simulink model "cube_controller"  (R2023b)
settings: Solver=VariableStepAuto  StartTime=0.0  StopTime=10.0  RelTol=1e-3
settings Model: Creator=charl  LastModifiedBy=charl

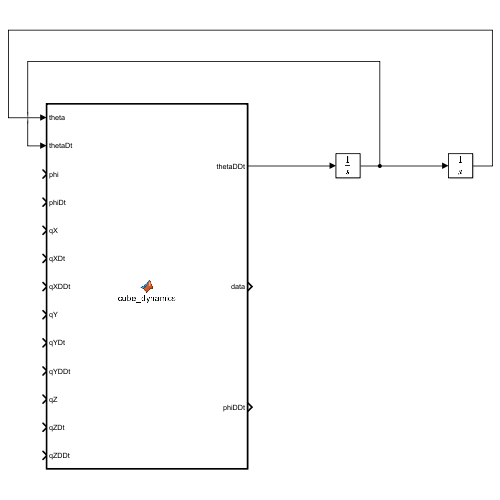
[thumbnail: Simulink's stored preview of the top-level diagram]
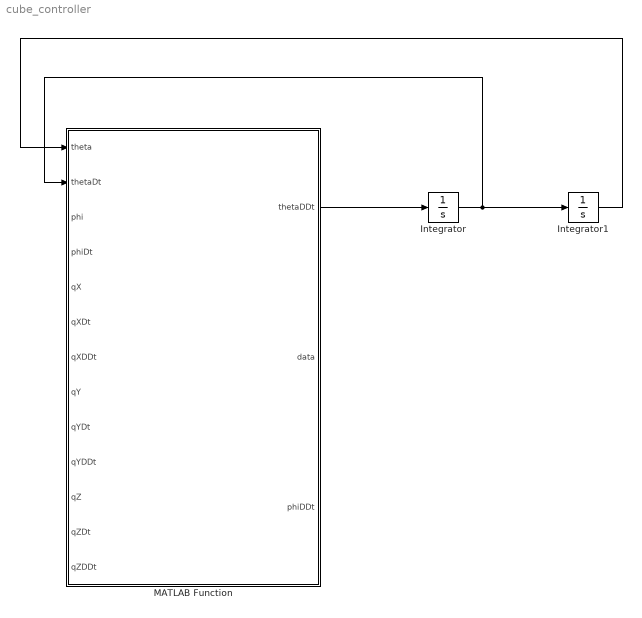
== system cube_controller ==
  Integrator : Integrator
  Integrator1 : Integrator
  MATLAB Function : MATLAB Function  TreatAsAtomicUnit=on
  wires:
  MATLAB Function/1(thetaDDt) -> Integrator/1
  Integrator/1 -> Integrator1/1, MATLAB Function/2(thetaDt)
  Integrator1/1 -> MATLAB Function/1(theta)

== matlab function cube_controller/MATLAB Function ==
  data: theta input; thetaDt input; thetaDDt output; data output; phi input; phiDt input; qX input; qXDt input; qXDDt input; qY input; qYDt input; qYDDt input; qZ input; qZDt input; qZDDt input; phiDDt output
function [thetaDDt, data, phiDDt]= cube_dynamics(theta, thetaDt, phi, phiDt, qX, qXDt, qXDDt, qY, qYDt, qYDDt, qZ, qZDt, qZDDt)


thetaDDt = -((RXIXY*sin(theta)*cos(phi+qX)+(RZIXY*cos(qZ)-RZIYY*sin(qZ))*(sin(qZ)*cos(theta)+sin(theta)*cos(phi)*cos(qZ))-RXIXZ*sin(  ...
theta)*sin(phi+qX)-(CIXX+RXIXX+mR*RCMZ^2+2*mR*(RCMY^2+1.5*RCMX^2))*cos(theta)-(RYIXZ*cos(qY)+RYIZZ*sin(qY))*(sin(qY)*cos(theta)+sin(  ...
phi)*sin(theta)*cos(qY))-(RYIXX*cos(qY)+RYIXZ*sin(qY))*(cos(qY)*cos(theta)-sin(phi)*sin(qY)*sin(theta))-(RZIXX*cos(qZ)-RZIXY*sin(  ...
qZ))*(cos(qZ)*cos(theta)-sin(qZ)*sin(theta)*cos(phi))-sin(phi)*sin(theta)*(CIXZ+mR*RCMX*RCMY+mR*RCMX^2+mR*RCMY*RCMZ+RZIXZ*cos(qZ)-  ...
RZIYZ*sin(qZ))-sin(theta)*cos(phi)*(mR*RCMX*RCMY+mR*RCMX*RCMZ+mR*RCMY*RCMZ-CIXY-RYIXY*cos(qY)-RYIYZ*sin(qY)))*(g*((mC*CCMZ+mR*RCMX+  ...
mR*RCMY+mR*RCMZ)*cos(theta)-(mC*CCMY+mR*RCMY+2*mR*RCMX)*sin(phi)*sin(theta)-(mC*CCMX+mR*RCMX+mR*RCMY+mR*RCMZ)*sin(theta)*cos(phi))+  ...
cos(phi+qX)*(2*RXIYZ*cos(phi+qX)*thetaDt*(phiDt+qXDt)+(phiDt+qXDt)*(RXIXY*(phiDt+qXDt)+2*RXIYY*sin(phi+qX)*thetaDt)+RXIXZ*qXDDt)+  ...
sin(qY)*cos(phi)*(RYIXX*sin(qY)*phiDt*qYDt+2*RYIXX*cos(phi)*cos(qY)*qYDt*thetaDt+2*RYIXZ*sin(qY)*cos(phi)*qYDt*thetaDt+4*RYIXZ*sin(  ...
phi)*cos(qY)*phiDt*thetaDt-4*RYIXZ*cos(qY)*phiDt*qYDt-2*RYIXY*cos(phi)*phiDt*thetaDt-2*RYIXX*sin(phi)*sin(qY)*phiDt*thetaDt-qYDt*(  ...
RYIYZ*qYDt+RYIZZ*sin(qY)*phiDt+2*RYIYZ*sin(phi)*thetaDt+2*RYIZZ*cos(phi)*cos(qY)*thetaDt)-RYIXY*qYDDt)-sin(phi+qX)*(2*RXIYZ*sin(phi+  ...
qX)*thetaDt*(phiDt+qXDt)+(phiDt+qXDt)*(RXIXZ*(phiDt+qXDt)+2*RXIZZ*cos(phi+qX)*thetaDt)-RXIXY*qXDDt)-cos(phi)*cos(qY)*(qYDt*(  ...
RYIXY*qYDt+RYIXX*cos(qY)*phiDt)+2*RYIXZ*cos(phi)*cos(qY)*qYDt*thetaDt-RYIZZ*cos(qY)*phiDt*qYDt-RYIYZ*qYDDt)-sin(phi)*cos(qZ)*(  ...
RZIYY*cos(qZ)*phiDt*qZDt+2*RZIXY*sin(qZ)*phiDt*qZDt+RZIYY*sin(phi)*sin(qZ)*qZDt*thetaDt-RZIXY*sin(phi)*cos(qZ)*qZDt*thetaDt-  ...
RZIYY*cos(phi)*cos(qZ)*phiDt*thetaDt-(qZDt+cos(phi)*thetaDt)*(RZIXZ*qZDt+RZIXX*cos(qZ)*phiDt+RZIXZ*cos(phi)*thetaDt+RZIXX*sin(phi)*  ...
sin(qZ)*thetaDt+RZIXY*sin(phi)*cos(qZ)*thetaDt)-RZIYZ*qZDDt)-sin(phi)*sin(qZ)*(RZIXX*sin(qZ)*phiDt*qZDt+RZIXY*sin(phi)*sin(qZ)*qZDt*  ...
thetaDt-2*RZIXY*cos(phi)*cos(qZ)*phiDt*thetaDt-RZIXX*sin(phi)*cos(qZ)*qZDt*thetaDt-RZIXX*sin(qZ)*cos(phi)*phiDt*thetaDt-(qZDt+cos(  ...
phi)*thetaDt)*(RZIYY*sin(qZ)*phiDt-RZIYZ*qZDt-2*RZIXY*cos(qZ)*phiDt-RZIYZ*cos(phi)*thetaDt-RZIXY*sin(phi)*sin(qZ)*thetaDt-RZIYY*sin(  ...
phi)*cos(qZ)*thetaDt)-RZIXZ*qZDDt)-sin(phi)*(2*RYIXY*cos(phi)*cos(qY)*qYDt*thetaDt+cos(qY)*phiDt*(RYIXZ*cos(qY)*phiDt+RYIZZ*sin(qY)*  ...
phiDt+2*RYIYZ*sin(phi)*thetaDt+2*RYIZZ*cos(phi)*cos(qY)*thetaDt)-2*CIYY*cos(phi)*phiDt*thetaDt-2*RYIYY*cos(phi)*phiDt*thetaDt-2*  ...
RYIXY*sin(phi)*sin(qY)*phiDt*thetaDt-sin(qY)*(RYIXX*cos(qY)+RYIXZ*sin(qY))*phiDt^2-phiDt*(RZIYZ*sin(qZ)*phiDt-CIXZ*phiDt-RZIZZ*qZDt-  ...
2*CIYZ*sin(phi)*thetaDt-2*CIZZ*cos(phi)*thetaDt-2*RZIZZ*cos(phi)*thetaDt-RZIXZ*cos(qZ)*phiDt-2*RZIXZ*sin(phi)*sin(qZ)*thetaDt-2*  ...
RZIYZ*sin(phi)*cos(qZ)*thetaDt-mR*RCMX*(RCMX*phiDt+4*RCMY*sin(phi)*thetaDt)-mR*(RCMY*RCMZ*phiDt-2*RCMX^2*cos(phi)*thetaDt)-mR*(RCMX*  ...
RCMY*phiDt+2*RCMZ*(RCMX*sin(phi)+RCMZ*cos(phi))*thetaDt))-RYIYY*qYDDt)-cos(phi)*(RZIXZ*sin(qZ)*phiDt*qZDt+RZIYZ*cos(qZ)*phiDt*qZDt+  ...
RZIYZ*sin(phi)*sin(qZ)*qZDt*thetaDt+(cos(qZ)*phiDt+sin(phi)*sin(qZ)*thetaDt)*(RZIYY*sin(qZ)*phiDt-RZIYZ*qZDt-RZIXY*cos(qZ)*phiDt-  ...
RZIYZ*cos(phi)*thetaDt-RZIXY*sin(phi)*sin(qZ)*thetaDt-RZIYY*sin(phi)*cos(qZ)*thetaDt)+(sin(qZ)*phiDt-sin(phi)*cos(qZ)*thetaDt)*(  ...
RZIXY*sin(qZ)*phiDt-RZIXZ*qZDt-RZIXX*cos(qZ)*phiDt-RZIXZ*cos(phi)*thetaDt-RZIXX*sin(phi)*sin(qZ)*thetaDt-RZIXY*sin(phi)*cos(qZ)*  ...
thetaDt)-2*CIYZ*cos(phi)*phiDt*thetaDt-RZIXZ*sin(phi)*cos(qZ)*qZDt*thetaDt-RZIXZ*sin(qZ)*cos(phi)*phiDt*thetaDt-RZIYZ*cos(phi)*cos(  ...
qZ)*phiDt*thetaDt-phiDt*(CIXY*phiDt+RYIYY*qYDt+RYIXY*cos(qY)*phiDt+RYIYZ*sin(qY)*phiDt+2*RYIYZ*cos(phi)*cos(qY)*thetaDt-mR*RCMX*RCMY*  ...
phiDt-mR*RCMX*(RCMZ*phiDt-4*RCMY*cos(phi)*thetaDt)-mR*RCMZ*(RCMY*phiDt-2*RCMX*cos(phi)*thetaDt))-RZIZZ*qZDDt))+(RXIXY*sin(phi+qX)+  ...
RXIXZ*cos(phi+qX)+cos(phi)*cos(qY)*(RYIXZ*cos(qY)+RYIZZ*sin(qY))+sin(phi)*sin(qZ)*(RZIXX*cos(qZ)-RZIXY*sin(qZ))+sin(phi)*cos(qZ)*(  ...
RZIXY*cos(qZ)-RZIYY*sin(qZ))+cos(phi)*(CIXZ+mR*RCMX*RCMY+mR*RCMX^2+mR*RCMY*RCMZ+RZIXZ*cos(qZ)-RZIYZ*sin(qZ))-sin(qY)*cos(phi)*(  ...
RYIXX*cos(qY)+RYIXZ*sin(qY))-sin(phi)*(mR*RCMX*RCMY+mR*RCMX*RCMZ+mR*RCMY*RCMZ-CIXY-RYIXY*cos(qY)-RYIYZ*sin(qY)))*(g*((mC*CCMY+mR*  ...
RCMY+2*mR*RCMX)*cos(phi)-(mC*CCMX+mR*RCMX+mR*RCMY+mR*RCMZ)*sin(phi))+sin(theta)*thetaDt*(mR*RCMZ*(RCMX*sin(phi)-RCMY*cos(phi))*  ...
thetaDt-CIXX*phiDt-RXIXX*(phiDt+qXDt)-CIXY*sin(phi)*thetaDt-CIXZ*cos(phi)*thetaDt-RXIXY*sin(phi+qX)*thetaDt-RXIXZ*cos(phi+qX)*  ...
thetaDt-2*mR*(RCMY^2+1.5*RCMX^2)*phiDt-mR*RCMX*(RCMX*cos(phi)-RCMY*sin(phi))*thetaDt-mR*(RCMZ^2*phiDt+RCMY*(RCMX*cos(phi)-RCMZ*sin(  ...
phi))*thetaDt))+sin(theta)*cos(phi+qX)*(4*RXIYZ*sin(phi+qX)*thetaDt*(phiDt+qXDt)+(phiDt+qXDt)*(RXIXZ*(phiDt+qXDt)+RXIZZ*cos(phi+qX)*  ...
thetaDt)-RXIYY*cos(phi+qX)*thetaDt*(phiDt+qXDt)-RXIXY*qXDDt)+(sin(qZ)*cos(theta)+sin(theta)*cos(phi)*cos(qZ))*(RZIXY*sin(qZ)*  ...
phiDt*qZDt+RZIYY*cos(qZ)*phiDt*qZDt+RZIYZ*sin(phi)*phiDt*thetaDt+RZIYY*sin(phi)*sin(qZ)*qZDt*thetaDt+(qZDt+cos(phi)*thetaDt)*(  ...
RZIXY*sin(qZ)*phiDt-RZIXZ*qZDt-RZIXX*cos(qZ)*phiDt-RZIXZ*cos(phi)*thetaDt-RZIXX*sin(phi)*sin(qZ)*thetaDt-RZIXY*sin(phi)*cos(qZ)*  ...
thetaDt)-RZIXY*sin(phi)*cos(qZ)*qZDt*thetaDt-RZIXY*sin(qZ)*cos(phi)*phiDt*thetaDt-RZIYY*cos(phi)*cos(qZ)*phiDt*thetaDt-RZIYZ*  ...
qZDDt)+sin(theta)*cos(phi)*(RYIXY*sin(qY)*phiDt*qYDt+RYIXY*cos(phi)*cos(qY)*qYDt*thetaDt+RYIYZ*sin(qY)*cos(phi)*qYDt*thetaDt+(sin(  ...
qY)*phiDt+cos(phi)*cos(qY)*thetaDt)*(RYIXX*sin(qY)*cos(phi)*thetaDt-RYIXY*qYDt-RYIXX*cos(qY)*phiDt-RYIXY*sin(phi)*thetaDt-RYIXZ*sin(  ...
qY)*phiDt-RYIXZ*cos(phi)*cos(qY)*thetaDt)-CIYY*cos(phi)*phiDt*thetaDt-RYIYY*cos(phi)*phiDt*thetaDt-RYIYZ*cos(qY)*phiDt*qYDt-(cos(  ...
qY)*phiDt-sin(qY)*cos(phi)*thetaDt)*(RYIXZ*sin(qY)*cos(phi)*thetaDt-RYIYZ*qYDt-RYIXZ*cos(qY)*phiDt-RYIYZ*sin(phi)*thetaDt-RYIZZ*sin(  ...
qY)*phiDt-RYIZZ*cos(phi)*cos(qY)*thetaDt)-phiDt*(RZIYZ*sin(qZ)*phiDt-CIXZ*phiDt-RZIZZ*qZDt-mR*RCMX^2*phiDt-CIZZ*cos(phi)*thetaDt-  ...
RZIXZ*cos(qZ)*phiDt-RZIZZ*cos(phi)*thetaDt-mR*(RCMX*RCMY*phiDt+RCMZ^2*cos(phi)*thetaDt)-mR*(RCMY*RCMZ*phiDt-RCMX^2*cos(phi)*  ...
thetaDt))-RYIYY*qYDDt)-sin(theta)*sin(phi+qX)*(RXIZZ*sin(phi+qX)*thetaDt*(phiDt+qXDt)-(phiDt+qXDt)*(RXIXY*(phiDt+qXDt)+RXIYY*sin(  ...
phi+qX)*thetaDt)-RXIXZ*qXDDt)-(sin(qY)*cos(theta)+sin(phi)*sin(theta)*cos(qY))*(RYIXZ*sin(qY)*phiDt*qYDt+RYIXZ*cos(phi)*cos(qY)*qYDt*  ...
thetaDt+RYIZZ*sin(phi)*cos(qY)*phiDt*thetaDt+RYIZZ*sin(qY)*cos(phi)*qYDt*thetaDt-RYIYZ*cos(phi)*phiDt*thetaDt-RYIZZ*cos(qY)*  ...
phiDt*qYDt-RYIXZ*sin(phi)*sin(qY)*phiDt*thetaDt-(qYDt+sin(phi)*thetaDt)*(RYIXX*sin(qY)*cos(phi)*thetaDt-RYIXY*qYDt-RYIXX*cos(qY)*  ...
phiDt-RYIXY*sin(phi)*thetaDt-RYIXZ*sin(qY)*phiDt-RYIXZ*cos(phi)*cos(qY)*thetaDt)-RYIYZ*qYDDt)-(cos(qY)*cos(theta)-sin(phi)*sin(qY)*  ...
sin(theta))*(RYIXX*sin(qY)*phiDt*qYDt+RYIXX*cos(phi)*cos(qY)*qYDt*thetaDt+RYIXZ*sin(phi)*cos(qY)*phiDt*thetaDt+RYIXZ*sin(qY)*cos(  ...
phi)*qYDt*thetaDt+(qYDt+sin(phi)*thetaDt)*(RYIXZ*sin(qY)*cos(phi)*thetaDt-RYIYZ*qYDt-RYIXZ*cos(qY)*phiDt-RYIYZ*sin(phi)*thetaDt-  ...
RYIZZ*sin(qY)*phiDt-RYIZZ*cos(phi)*cos(qY)*thetaDt)-RYIXY*cos(phi)*phiDt*thetaDt-RYIXZ*cos(qY)*phiDt*qYDt-RYIXX*sin(phi)*sin(qY)*  ...
phiDt*thetaDt-RYIXY*qYDDt)-(cos(qZ)*cos(theta)-sin(qZ)*sin(theta)*cos(phi))*(RZIXX*sin(qZ)*phiDt*qZDt+RZIXY*cos(qZ)*phiDt*qZDt+  ...
RZIXZ*sin(phi)*phiDt*thetaDt+RZIXY*sin(phi)*sin(qZ)*qZDt*thetaDt-RZIXX*sin(phi)*cos(qZ)*qZDt*thetaDt-RZIXX*sin(qZ)*cos(phi)*  ...
phiDt*thetaDt-RZIXY*cos(phi)*cos(qZ)*phiDt*thetaDt-(qZDt+cos(phi)*thetaDt)*(RZIYY*sin(qZ)*phiDt-RZIYZ*qZDt-RZIXY*cos(qZ)*phiDt-  ...
RZIYZ*cos(phi)*thetaDt-RZIXY*sin(phi)*sin(qZ)*thetaDt-RZIYY*sin(phi)*cos(qZ)*thetaDt)-RZIXZ*qZDDt)-cos(theta)*(sin(phi)*thetaDt*(  ...
RZIYZ*sin(qZ)*phiDt-RZIZZ*qZDt-CIYZ*sin(phi)*thetaDt-CIZZ*cos(phi)*thetaDt-RZIXZ*cos(qZ)*phiDt-RZIZZ*cos(phi)*thetaDt-2*mR*RCMX*RCMY*  ...
sin(phi)*thetaDt-RZIXZ*sin(phi)*sin(qZ)*thetaDt-RZIYZ*sin(phi)*cos(qZ)*thetaDt-mR*RCMZ*(RCMX*sin(phi)+RCMZ*cos(phi))*thetaDt)-(sin(  ...
phi+qX)*(RXIYZ*sin(phi+qX)+RXIZZ*cos(phi+qX))-cos(phi+qX)*(RXIYY*sin(phi+qX)+RXIYZ*cos(phi+qX)))*thetaDt^2-cos(phi)*thetaDt*(  ...
RYIXY*sin(qY)*cos(phi)*thetaDt-RYIYY*qYDt-CIYY*sin(phi)*thetaDt-CIYZ*cos(phi)*thetaDt-RYIXY*cos(qY)*phiDt-RYIYY*sin(phi)*thetaDt-  ...
RYIYZ*sin(qY)*phiDt-2*mR*RCMX*RCMY*cos(phi)*thetaDt-mR*RCMX*RCMZ*cos(phi)*thetaDt-mR*RCMX^2*sin(phi)*thetaDt-RYIYZ*cos(phi)*cos(qY)*  ...
thetaDt)-RXIXX*qXDDt)-sin(phi)*sin(theta)*(CIZZ*sin(phi)*phiDt*thetaDt+RZIXZ*sin(qZ)*phiDt*qZDt+RZIYZ*cos(qZ)*phiDt*qZDt+RZIZZ*sin(  ...
phi)*phiDt*thetaDt+mR*RCMZ^2*sin(phi)*phiDt*thetaDt+RZIYZ*sin(phi)*sin(qZ)*qZDt*thetaDt+(cos(qZ)*phiDt+sin(phi)*sin(qZ)*thetaDt)*(  ...
RZIYY*sin(qZ)*phiDt-RZIYZ*qZDt-RZIXY*cos(qZ)*phiDt-RZIYZ*cos(phi)*thetaDt-RZIXY*sin(phi)*sin(qZ)*thetaDt-RZIYY*sin(phi)*cos(qZ)*  ...
thetaDt)+(sin(qZ)*phiDt-sin(phi)*cos(qZ)*thetaDt)*(RZIXY*sin(qZ)*phiDt-RZIXZ*qZDt-RZIXX*cos(qZ)*phiDt-RZIXZ*cos(phi)*thetaDt-  ...
RZIXX*sin(phi)*sin(qZ)*thetaDt-RZIXY*sin(phi)*cos(qZ)*thetaDt)-4*CIYZ*cos(phi)*phiDt*thetaDt-2*RZIXZ*sin(qZ)*cos(phi)*phiDt*  ...
thetaDt-2*RZIYZ*cos(phi)*cos(qZ)*phiDt*thetaDt-RZIXZ*sin(phi)*cos(qZ)*qZDt*thetaDt-phiDt*(CIXY*phiDt+RYIYY*qYDt+CIYY*sin(phi)*  ...
thetaDt+RYIXY*cos(qY)*phiDt+RYIYY*sin(phi)*thetaDt+RYIYZ*sin(qY)*phiDt+2*RYIYZ*cos(phi)*cos(qY)*thetaDt-2*RYIXY*sin(qY)*cos(phi)*  ...
thetaDt-mR*RCMX*(RCMY*phiDt-RCMX*sin(phi)*thetaDt)-mR*RCMX*(RCMZ*phiDt-8*RCMY*cos(phi)*thetaDt)-mR*RCMZ*(RCMY*phiDt-4*RCMX*cos(phi)*  ...
thetaDt))-RZIZZ*qZDDt)))/((2*mR*RCMY^2+mR*(RCMX^2+RCMZ^2)+RXIYY*sin(phi+qX)^2+RYIZZ*cos(phi)^2*cos(qY)^2+RZIXX*sin(phi)^2*sin(qZ)^2+  ...
cos(phi+qX)*(RXIZZ*cos(phi+qX)+2*RXIYZ*sin(phi+qX))+cos(qZ)*sin(phi)^2*(RZIYY*cos(qZ)+2*RZIXY*sin(qZ))+sin(qY)*cos(phi)*(RYIXX*sin(  ...
qY)*cos(phi)-2*RYIXY*sin(phi)-2*RYIXZ*cos(phi)*cos(qY))+cos(phi)*(CIZZ*cos(phi)+RZIZZ*cos(phi)+mR*RCMX^2*cos(phi)+mR*RCMZ^2*cos(phi)+  ...
2*RZIXZ*sin(phi)*sin(qZ)+2*RZIYZ*sin(phi)*cos(qZ))+sin(phi)*(CIYY*sin(phi)+RYIYY*sin(phi)+2*CIYZ*cos(phi)+2*mR*RCMX*RCMZ*cos(phi)+  ...
2*mR*RCMX^2*sin(phi)+4*mR*RCMX*RCMY*cos(phi)+2*RYIYZ*cos(phi)*cos(qY)))*(RXIXY*sin(theta)*cos(phi+qX)+(RZIXY*cos(qZ)-RZIYY*sin(qZ))*(  ...
sin(qZ)*cos(theta)+sin(theta)*cos(phi)*cos(qZ))-RXIXZ*sin(theta)*sin(phi+qX)-(CIXX+RXIXX+mR*RCMZ^2+2*mR*(RCMY^2+1.5*RCMX^2))*cos(  ...
theta)-(RYIXZ*cos(qY)+RYIZZ*sin(qY))*(sin(qY)*cos(theta)+sin(phi)*sin(theta)*cos(qY))-(RYIXX*cos(qY)+RYIXZ*sin(qY))*(cos(qY)*cos(  ...
theta)-sin(phi)*sin(qY)*sin(theta))-(RZIXX*cos(qZ)-RZIXY*sin(qZ))*(cos(qZ)*cos(theta)-sin(qZ)*sin(theta)*cos(phi))-sin(phi)*sin(  ...
theta)*(CIXZ+mR*RCMX*RCMY+mR*RCMX^2+mR*RCMY*RCMZ+RZIXZ*cos(qZ)-RZIYZ*sin(qZ))-sin(theta)*cos(phi)*(mR*RCMX*RCMY+mR*RCMX*RCMZ+mR*RCMY*  ...
RCMZ-CIXY-RYIXY*cos(qY)-RYIYZ*sin(qY)))+(RXIXY*sin(phi+qX)+RXIXZ*cos(phi+qX)+cos(phi)*cos(qY)*(RYIXZ*cos(qY)+RYIZZ*sin(qY))+sin(phi)*  ...
sin(qZ)*(RZIXX*cos(qZ)-RZIXY*sin(qZ))+sin(phi)*cos(qZ)*(RZIXY*cos(qZ)-RZIYY*sin(qZ))+cos(phi)*(CIXZ+mR*RCMX*RCMY+mR*RCMX^2+mR*RCMY*  ...
RCMZ+RZIXZ*cos(qZ)-RZIYZ*sin(qZ))-sin(qY)*cos(phi)*(RYIXX*cos(qY)+RYIXZ*sin(qY))-sin(phi)*(mR*RCMX*RCMY+mR*RCMX*RCMZ+mR*RCMY*RCMZ-  ...
CIXY-RYIXY*cos(qY)-RYIYZ*sin(qY)))*(sin(theta)*sin(phi+qX)*(RXIYZ*sin(phi+qX)+RXIZZ*cos(phi+qX))+(cos(qZ)*cos(theta)-sin(qZ)*sin(  ...
theta)*cos(phi))*(RZIXZ*cos(phi)+RZIXX*sin(phi)*sin(qZ)+RZIXY*sin(phi)*cos(qZ))+sin(theta)*cos(phi)*(RYIXY*sin(qY)*cos(phi)-CIYY*  ...
sin(phi)-CIYZ*cos(phi)-RYIYY*sin(phi)-2*mR*RCMX*RCMY*cos(phi)-mR*RCMX*RCMZ*cos(phi)-RYIYZ*cos(phi)*cos(qY))+cos(theta)*(CIXY*sin(  ...
phi)+CIXZ*cos(phi)+RXIXY*sin(phi+qX)+RXIXZ*cos(phi+qX)+mR*RCMX*(RCMX*cos(phi)-RCMY*sin(phi))+mR*RCMY*(RCMX*cos(phi)-RCMZ*sin(phi))-  ...
mR*RCMZ*(RCMX*sin(phi)-RCMY*cos(phi)))-sin(theta)*cos(phi+qX)*(RXIYY*sin(phi+qX)+RXIYZ*cos(phi+qX))-(sin(qZ)*cos(theta)+sin(  ...
theta)*cos(phi)*cos(qZ))*(RZIYZ*cos(phi)+RZIXY*sin(phi)*sin(qZ)+RZIYY*sin(phi)*cos(qZ))-(sin(qY)*cos(theta)+sin(phi)*sin(theta)*cos(  ...
qY))*(RYIXZ*sin(qY)*cos(phi)-RYIYZ*sin(phi)-RYIZZ*cos(phi)*cos(qY))-(cos(qY)*cos(theta)-sin(phi)*sin(qY)*sin(theta))*(RYIXX*sin(qY)*  ...
cos(phi)-RYIXY*sin(phi)-RYIXZ*cos(phi)*cos(qY))-sin(phi)*sin(theta)*(mR*RCMX^2*cos(phi)-CIYZ*sin(phi)-CIZZ*cos(phi)-RZIZZ*cos(phi)-  ...
2*mR*RCMX*RCMY*sin(phi)-RZIXZ*sin(phi)*sin(qZ)-RZIYZ*sin(phi)*cos(qZ)-mR*RCMZ*(RCMX*sin(phi)+RCMZ*cos(phi)))));
phiDDt = -((sin(theta)*sin(phi+qX)*(RXIYZ*sin(phi+qX)+RXIZZ*cos(phi+qX))+(cos(qZ)*cos(theta)-sin(qZ)*sin(theta)*cos(phi))*(RZIXZ*  ...
cos(phi)+RZIXX*sin(phi)*sin(qZ)+RZIXY*sin(phi)*cos(qZ))+sin(theta)*cos(phi)*(RYIXY*sin(qY)*cos(phi)-CIYY*sin(phi)-CIYZ*cos(phi)-  ...
RYIYY*sin(phi)-2*mR*RCMX*RCMY*cos(phi)-mR*RCMX*RCMZ*cos(phi)-RYIYZ*cos(phi)*cos(qY))+cos(theta)*(CIXY*sin(phi)+CIXZ*cos(phi)+  ...
RXIXY*sin(phi+qX)+RXIXZ*cos(phi+qX)+mR*RCMX*(RCMX*cos(phi)-RCMY*sin(phi))+mR*RCMY*(RCMX*cos(phi)-RCMZ*sin(phi))-mR*RCMZ*(RCMX*sin(  ...
phi)-RCMY*cos(phi)))-sin(theta)*cos(phi+qX)*(RXIYY*sin(phi+qX)+RXIYZ*cos(phi+qX))-(sin(qZ)*cos(theta)+sin(theta)*cos(phi)*cos(qZ))*(  ...
RZIYZ*cos(phi)+RZIXY*sin(phi)*sin(qZ)+RZIYY*sin(phi)*cos(qZ))-(sin(qY)*cos(theta)+sin(phi)*sin(theta)*cos(qY))*(RYIXZ*sin(qY)*cos(  ...
phi)-RYIYZ*sin(phi)-RYIZZ*cos(phi)*cos(qY))-(cos(qY)*cos(theta)-sin(phi)*sin(qY)*sin(theta))*(RYIXX*sin(qY)*cos(phi)-RYIXY*sin(phi)-  ...
RYIXZ*cos(phi)*cos(qY))-sin(phi)*sin(theta)*(mR*RCMX^2*cos(phi)-CIYZ*sin(phi)-CIZZ*cos(phi)-RZIZZ*cos(phi)-2*mR*RCMX*RCMY*sin(phi)-  ...
RZIXZ*sin(phi)*sin(qZ)-RZIYZ*sin(phi)*cos(qZ)-mR*RCMZ*(RCMX*sin(phi)+RCMZ*cos(phi))))*(g*((mC*CCMZ+mR*RCMX+mR*RCMY+mR*RCMZ)*cos(  ...
theta)-(mC*CCMY+mR*RCMY+2*mR*RCMX)*sin(phi)*sin(theta)-(mC*CCMX+mR*RCMX+mR*RCMY+mR*RCMZ)*sin(theta)*cos(phi))+cos(phi+qX)*(2*  ...
RXIYZ*cos(phi+qX)*thetaDt*(phiDt+qXDt)+(phiDt+qXDt)*(RXIXY*(phiDt+qXDt)+2*RXIYY*sin(phi+qX)*thetaDt)+RXIXZ*qXDDt)+sin(qY)*cos(phi)*(  ...
RYIXX*sin(qY)*phiDt*qYDt+2*RYIXX*cos(phi)*cos(qY)*qYDt*thetaDt+2*RYIXZ*sin(qY)*cos(phi)*qYDt*thetaDt+4*RYIXZ*sin(phi)*cos(qY)*  ...
phiDt*thetaDt-4*RYIXZ*cos(qY)*phiDt*qYDt-2*RYIXY*cos(phi)*phiDt*thetaDt-2*RYIXX*sin(phi)*sin(qY)*phiDt*thetaDt-qYDt*(RYIYZ*qYDt+  ...
RYIZZ*sin(qY)*phiDt+2*RYIYZ*sin(phi)*thetaDt+2*RYIZZ*cos(phi)*cos(qY)*thetaDt)-RYIXY*qYDDt)-sin(phi+qX)*(2*RXIYZ*sin(phi+qX)*  ...
thetaDt*(phiDt+qXDt)+(phiDt+qXDt)*(RXIXZ*(phiDt+qXDt)+2*RXIZZ*cos(phi+qX)*thetaDt)-RXIXY*qXDDt)-cos(phi)*cos(qY)*(qYDt*(RYIXY*qYDt+  ...
RYIXX*cos(qY)*phiDt)+2*RYIXZ*cos(phi)*cos(qY)*qYDt*thetaDt-RYIZZ*cos(qY)*phiDt*qYDt-RYIYZ*qYDDt)-sin(phi)*cos(qZ)*(RZIYY*cos(qZ)*  ...
phiDt*qZDt+2*RZIXY*sin(qZ)*phiDt*qZDt+RZIYY*sin(phi)*sin(qZ)*qZDt*thetaDt-RZIXY*sin(phi)*cos(qZ)*qZDt*thetaDt-RZIYY*cos(phi)*cos(  ...
qZ)*phiDt*thetaDt-(qZDt+cos(phi)*thetaDt)*(RZIXZ*qZDt+RZIXX*cos(qZ)*phiDt+RZIXZ*cos(phi)*thetaDt+RZIXX*sin(phi)*sin(qZ)*thetaDt+  ...
RZIXY*sin(phi)*cos(qZ)*thetaDt)-RZIYZ*qZDDt)-sin(phi)*sin(qZ)*(RZIXX*sin(qZ)*phiDt*qZDt+RZIXY*sin(phi)*sin(qZ)*qZDt*thetaDt-2*  ...
RZIXY*cos(phi)*cos(qZ)*phiDt*thetaDt-RZIXX*sin(phi)*cos(qZ)*qZDt*thetaDt-RZIXX*sin(qZ)*cos(phi)*phiDt*thetaDt-(qZDt+cos(phi)*  ...
thetaDt)*(RZIYY*sin(qZ)*phiDt-RZIYZ*qZDt-2*RZIXY*cos(qZ)*phiDt-RZIYZ*cos(phi)*thetaDt-RZIXY*sin(phi)*sin(qZ)*thetaDt-RZIYY*sin(phi)*  ...
cos(qZ)*thetaDt)-RZIXZ*qZDDt)-sin(phi)*(2*RYIXY*cos(phi)*cos(qY)*qYDt*thetaDt+cos(qY)*phiDt*(RYIXZ*cos(qY)*phiDt+RYIZZ*sin(qY)*  ...
phiDt+2*RYIYZ*sin(phi)*thetaDt+2*RYIZZ*cos(phi)*cos(qY)*thetaDt)-2*CIYY*cos(phi)*phiDt*thetaDt-2*RYIYY*cos(phi)*phiDt*thetaDt-2*  ...
RYIXY*sin(phi)*sin(qY)*phiDt*thetaDt-sin(qY)*(RYIXX*cos(qY)+RYIXZ*sin(qY))*phiDt^2-phiDt*(RZIYZ*sin(qZ)*phiDt-CIXZ*phiDt-RZIZZ*qZDt-  ...
2*CIYZ*sin(phi)*thetaDt-2*CIZZ*cos(phi)*thetaDt-2*RZIZZ*cos(phi)*thetaDt-RZIXZ*cos(qZ)*phiDt-2*RZIXZ*sin(phi)*sin(qZ)*thetaDt-2*  ...
RZIYZ*sin(phi)*cos(qZ)*thetaDt-mR*RCMX*(RCMX*phiDt+4*RCMY*sin(phi)*thetaDt)-mR*(RCMY*RCMZ*phiDt-2*RCMX^2*cos(phi)*thetaDt)-mR*(RCMX*  ...
RCMY*phiDt+2*RCMZ*(RCMX*sin(phi)+RCMZ*cos(phi))*thetaDt))-RYIYY*qYDDt)-cos(phi)*(RZIXZ*sin(qZ)*phiDt*qZDt+RZIYZ*cos(qZ)*phiDt*qZDt+  ...
RZIYZ*sin(phi)*sin(qZ)*qZDt*thetaDt+(cos(qZ)*phiDt+sin(phi)*sin(qZ)*thetaDt)*(RZIYY*sin(qZ)*phiDt-RZIYZ*qZDt-RZIXY*cos(qZ)*phiDt-  ...
RZIYZ*cos(phi)*thetaDt-RZIXY*sin(phi)*sin(qZ)*thetaDt-RZIYY*sin(phi)*cos(qZ)*thetaDt)+(sin(qZ)*phiDt-sin(phi)*cos(qZ)*thetaDt)*(  ...
RZIXY*sin(qZ)*phiDt-RZIXZ*qZDt-RZIXX*cos(qZ)*phiDt-RZIXZ*cos(phi)*thetaDt-RZIXX*sin(phi)*sin(qZ)*thetaDt-RZIXY*sin(phi)*cos(qZ)*  ...
thetaDt)-2*CIYZ*cos(phi)*phiDt*thetaDt-RZIXZ*sin(phi)*cos(qZ)*qZDt*thetaDt-RZIXZ*sin(qZ)*cos(phi)*phiDt*thetaDt-RZIYZ*cos(phi)*cos(  ...
qZ)*phiDt*thetaDt-phiDt*(CIXY*phiDt+RYIYY*qYDt+RYIXY*cos(qY)*phiDt+RYIYZ*sin(qY)*phiDt+2*RYIYZ*cos(phi)*cos(qY)*thetaDt-mR*RCMX*RCMY*  ...
phiDt-mR*RCMX*(RCMZ*phiDt-4*RCMY*cos(phi)*thetaDt)-mR*RCMZ*(RCMY*phiDt-2*RCMX*cos(phi)*thetaDt))-RZIZZ*qZDDt))-(2*mR*RCMY^2+mR*(RCMX^2+RCMZ^2)+  ...
RXIYY*sin(phi+qX)^2+RYIZZ*cos(phi)^2*cos(qY)^2+RZIXX*sin(phi)^2*sin(qZ)^2+cos(phi+qX)*(RXIZZ*cos(phi+qX)+2*RXIYZ*sin(phi+qX))+cos(  ...
qZ)*sin(phi)^2*(RZIYY*cos(qZ)+2*RZIXY*sin(qZ))+sin(qY)*cos(phi)*(RYIXX*sin(qY)*cos(phi)-2*RYIXY*sin(phi)-2*RYIXZ*cos(phi)*cos(qY))+  ...
cos(phi)*(CIZZ*cos(phi)+RZIZZ*cos(phi)+mR*RCMX^2*cos(phi)+mR*RCMZ^2*cos(phi)+2*RZIXZ*sin(phi)*sin(qZ)+2*RZIYZ*sin(phi)*cos(qZ))+sin(  ...
phi)*(CIYY*sin(phi)+RYIYY*sin(phi)+2*CIYZ*cos(phi)+2*mR*RCMX*RCMZ*cos(phi)+2*mR*RCMX^2*sin(phi)+4*mR*RCMX*RCMY*cos(phi)+2*RYIYZ*cos(  ...
phi)*cos(qY)))*(g*((mC*CCMY+mR*RCMY+2*mR*RCMX)*cos(phi)-(mC*CCMX+mR*RCMX+mR*RCMY+mR*RCMZ)*sin(phi))+sin(theta)*thetaDt*(mR*RCMZ*(  ...
RCMX*sin(phi)-RCMY*cos(phi))*thetaDt-CIXX*phiDt-RXIXX*(phiDt+qXDt)-CIXY*sin(phi)*thetaDt-CIXZ*cos(phi)*thetaDt-RXIXY*sin(phi+qX)*  ...
thetaDt-RXIXZ*cos(phi+qX)*thetaDt-2*mR*(RCMY^2+1.5*RCMX^2)*phiDt-mR*RCMX*(RCMX*cos(phi)-RCMY*sin(phi))*thetaDt-mR*(RCMZ^2*phiDt+RCMY*(  ...
RCMX*cos(phi)-RCMZ*sin(phi))*thetaDt))+sin(theta)*cos(phi+qX)*(4*RXIYZ*sin(phi+qX)*thetaDt*(phiDt+qXDt)+(phiDt+qXDt)*(RXIXZ*(  ...
phiDt+qXDt)+RXIZZ*cos(phi+qX)*thetaDt)-RXIYY*cos(phi+qX)*thetaDt*(phiDt+qXDt)-RXIXY*qXDDt)+(sin(qZ)*cos(theta)+sin(theta)*cos(phi)*  ...
cos(qZ))*(RZIXY*sin(qZ)*phiDt*qZDt+RZIYY*cos(qZ)*phiDt*qZDt+RZIYZ*sin(phi)*phiDt*thetaDt+RZIYY*sin(phi)*sin(qZ)*qZDt*thetaDt+(qZDt+  ...
cos(phi)*thetaDt)*(RZIXY*sin(qZ)*phiDt-RZIXZ*qZDt-RZIXX*cos(qZ)*phiDt-RZIXZ*cos(phi)*thetaDt-RZIXX*sin(phi)*sin(qZ)*thetaDt-  ...
RZIXY*sin(phi)*cos(qZ)*thetaDt)-RZIXY*sin(phi)*cos(qZ)*qZDt*thetaDt-RZIXY*sin(qZ)*cos(phi)*phiDt*thetaDt-RZIYY*cos(phi)*cos(qZ)*  ...
phiDt*thetaDt-RZIYZ*qZDDt)+sin(theta)*cos(phi)*(RYIXY*sin(qY)*phiDt*qYDt+RYIXY*cos(phi)*cos(qY)*qYDt*thetaDt+RYIYZ*sin(qY)*cos(phi)*  ...
qYDt*thetaDt+(sin(qY)*phiDt+cos(phi)*cos(qY)*thetaDt)*(RYIXX*sin(qY)*cos(phi)*thetaDt-RYIXY*qYDt-RYIXX*cos(qY)*phiDt-RYIXY*sin(phi)*  ...
thetaDt-RYIXZ*sin(qY)*phiDt-RYIXZ*cos(phi)*cos(qY)*thetaDt)-CIYY*cos(phi)*phiDt*thetaDt-RYIYY*cos(phi)*phiDt*thetaDt-RYIYZ*cos(qY)*  ...
phiDt*qYDt-(cos(qY)*phiDt-sin(qY)*cos(phi)*thetaDt)*(RYIXZ*sin(qY)*cos(phi)*thetaDt-RYIYZ*qYDt-RYIXZ*cos(qY)*phiDt-RYIYZ*sin(phi)*  ...
thetaDt-RYIZZ*sin(qY)*phiDt-RYIZZ*cos(phi)*cos(qY)*thetaDt)-phiDt*(RZIYZ*sin(qZ)*phiDt-CIXZ*phiDt-RZIZZ*qZDt-mR*RCMX^2*phiDt-CIZZ*  ...
cos(phi)*thetaDt-RZIXZ*cos(qZ)*phiDt-RZIZZ*cos(phi)*thetaDt-mR*(RCMX*RCMY*phiDt+RCMZ^2*cos(phi)*thetaDt)-mR*(RCMY*RCMZ*phiDt-RCMX^2*  ...
cos(phi)*thetaDt))-RYIYY*qYDDt)-sin(theta)*sin(phi+qX)*(RXIZZ*sin(phi+qX)*thetaDt*(phiDt+qXDt)-(phiDt+qXDt)*(RXIXY*(phiDt+qXDt)+  ...
RXIYY*sin(phi+qX)*thetaDt)-RXIXZ*qXDDt)-(sin(qY)*cos(theta)+sin(phi)*sin(theta)*cos(qY))*(RYIXZ*sin(qY)*phiDt*qYDt+RYIXZ*cos(phi)*  ...
cos(qY)*qYDt*thetaDt+RYIZZ*sin(phi)*cos(qY)*phiDt*thetaDt+RYIZZ*sin(qY)*cos(phi)*qYDt*thetaDt-RYIYZ*cos(phi)*phiDt*thetaDt-RYIZZ*  ...
cos(qY)*phiDt*qYDt-RYIXZ*sin(phi)*sin(qY)*phiDt*thetaDt-(qYDt+sin(phi)*thetaDt)*(RYIXX*sin(qY)*cos(phi)*thetaDt-RYIXY*qYDt-RYIXX*  ...
cos(qY)*phiDt-RYIXY*sin(phi)*thetaDt-RYIXZ*sin(qY)*phiDt-RYIXZ*cos(phi)*cos(qY)*thetaDt)-RYIYZ*qYDDt)-(cos(qY)*cos(theta)-sin(phi)*  ...
sin(qY)*sin(theta))*(RYIXX*sin(qY)*phiDt*qYDt+RYIXX*cos(phi)*cos(qY)*qYDt*thetaDt+RYIXZ*sin(phi)*cos(qY)*phiDt*thetaDt+RYIXZ*sin(  ...
qY)*cos(phi)*qYDt*thetaDt+(qYDt+sin(phi)*thetaDt)*(RYIXZ*sin(qY)*cos(phi)*thetaDt-RYIYZ*qYDt-RYIXZ*cos(qY)*phiDt-RYIYZ*sin(phi)*  ...
thetaDt-RYIZZ*sin(qY)*phiDt-RYIZZ*cos(phi)*cos(qY)*thetaDt)-RYIXY*cos(phi)*phiDt*thetaDt-RYIXZ*cos(qY)*phiDt*qYDt-RYIXX*sin(phi)*  ...
sin(qY)*phiDt*thetaDt-RYIXY*qYDDt)-(cos(qZ)*cos(theta)-sin(qZ)*sin(theta)*cos(phi))*(RZIXX*sin(qZ)*phiDt*qZDt+RZIXY*cos(qZ)*  ...
phiDt*qZDt+RZIXZ*sin(phi)*phiDt*thetaDt+RZIXY*sin(phi)*sin(qZ)*qZDt*thetaDt-RZIXX*sin(phi)*cos(qZ)*qZDt*thetaDt-RZIXX*sin(qZ)*cos(  ...
phi)*phiDt*thetaDt-RZIXY*cos(phi)*cos(qZ)*phiDt*thetaDt-(qZDt+cos(phi)*thetaDt)*(RZIYY*sin(qZ)*phiDt-RZIYZ*qZDt-RZIXY*cos(qZ)*  ...
phiDt-RZIYZ*cos(phi)*thetaDt-RZIXY*sin(phi)*sin(qZ)*thetaDt-RZIYY*sin(phi)*cos(qZ)*thetaDt)-RZIXZ*qZDDt)-cos(theta)*(sin(phi)*  ...
thetaDt*(RZIYZ*sin(qZ)*phiDt-RZIZZ*qZDt-CIYZ*sin(phi)*thetaDt-CIZZ*cos(phi)*thetaDt-RZIXZ*cos(qZ)*phiDt-RZIZZ*cos(phi)*thetaDt-2*  ...
mR*RCMX*RCMY*sin(phi)*thetaDt-RZIXZ*sin(phi)*sin(qZ)*thetaDt-RZIYZ*sin(phi)*cos(qZ)*thetaDt-mR*RCMZ*(RCMX*sin(phi)+RCMZ*cos(phi))*  ...
thetaDt)-(sin(phi+qX)*(RXIYZ*sin(phi+qX)+RXIZZ*cos(phi+qX))-cos(phi+qX)*(RXIYY*sin(phi+qX)+RXIYZ*cos(phi+qX)))*thetaDt^2-cos(phi)*  ...
thetaDt*(RYIXY*sin(qY)*cos(phi)*thetaDt-RYIYY*qYDt-CIYY*sin(phi)*thetaDt-CIYZ*cos(phi)*thetaDt-RYIXY*cos(qY)*phiDt-RYIYY*sin(phi)*  ...
thetaDt-RYIYZ*sin(qY)*phiDt-2*mR*RCMX*RCMY*cos(phi)*thetaDt-mR*RCMX*RCMZ*cos(phi)*thetaDt-mR*RCMX^2*sin(phi)*thetaDt-RYIYZ*cos(phi)*  ...
cos(qY)*thetaDt)-RXIXX*qXDDt)-sin(phi)*sin(theta)*(CIZZ*sin(phi)*phiDt*thetaDt+RZIXZ*sin(qZ)*phiDt*qZDt+RZIYZ*cos(qZ)*phiDt*qZDt+  ...
RZIZZ*sin(phi)*phiDt*thetaDt+mR*RCMZ^2*sin(phi)*phiDt*thetaDt+RZIYZ*sin(phi)*sin(qZ)*qZDt*thetaDt+(cos(qZ)*phiDt+sin(phi)*sin(qZ)*  ...
thetaDt)*(RZIYY*sin(qZ)*phiDt-RZIYZ*qZDt-RZIXY*cos(qZ)*phiDt-RZIYZ*cos(phi)*thetaDt-RZIXY*sin(phi)*sin(qZ)*thetaDt-RZIYY*sin(phi)*  ...
cos(qZ)*thetaDt)+(sin(qZ)*phiDt-sin(phi)*cos(qZ)*thetaDt)*(RZIXY*sin(qZ)*phiDt-RZIXZ*qZDt-RZIXX*cos(qZ)*phiDt-RZIXZ*cos(phi)*  ...
thetaDt-RZIXX*sin(phi)*sin(qZ)*thetaDt-RZIXY*sin(phi)*cos(qZ)*thetaDt)-4*CIYZ*cos(phi)*phiDt*thetaDt-2*RZIXZ*sin(qZ)*cos(phi)*  ...
phiDt*thetaDt-2*RZIYZ*cos(phi)*cos(qZ)*phiDt*thetaDt-RZIXZ*sin(phi)*cos(qZ)*qZDt*thetaDt-phiDt*(CIXY*phiDt+RYIYY*qYDt+CIYY*sin(phi)*  ...
thetaDt+RYIXY*cos(qY)*phiDt+RYIYY*sin(phi)*thetaDt+RYIYZ*sin(qY)*phiDt+2*RYIYZ*cos(phi)*cos(qY)*thetaDt-2*RYIXY*sin(qY)*cos(phi)*  ...
thetaDt-mR*RCMX*(RCMY*phiDt-RCMX*sin(phi)*thetaDt)-mR*RCMX*(RCMZ*phiDt-8*RCMY*cos(phi)*thetaDt)-mR*RCMZ*(RCMY*phiDt-4*RCMX*cos(phi)*  ...
thetaDt))-RZIZZ*qZDDt)))/((2*mR*RCMY^2+mR*(RCMX^2+RCMZ^2)+RXIYY*sin(phi+qX)^2+RYIZZ*cos(phi)^2*cos(qY)^2+RZIXX*sin(phi)^2*sin(qZ)^2+  ...
cos(phi+qX)*(RXIZZ*cos(phi+qX)+2*RXIYZ*sin(phi+qX))+cos(qZ)*sin(phi)^2*(RZIYY*cos(qZ)+2*RZIXY*sin(qZ))+sin(qY)*cos(phi)*(RYIXX*sin(  ...
qY)*cos(phi)-2*RYIXY*sin(phi)-2*RYIXZ*cos(phi)*cos(qY))+cos(phi)*(CIZZ*cos(phi)+RZIZZ*cos(phi)+mR*RCMX^2*cos(phi)+mR*RCMZ^2*cos(phi)+  ...
2*RZIXZ*sin(phi)*sin(qZ)+2*RZIYZ*sin(phi)*cos(qZ))+sin(phi)*(CIYY*sin(phi)+RYIYY*sin(phi)+2*CIYZ*cos(phi)+2*mR*RCMX*RCMZ*cos(phi)+  ...
2*mR*RCMX^2*sin(phi)+4*mR*RCMX*RCMY*cos(phi)+2*RYIYZ*cos(phi)*cos(qY)))*(RXIXY*sin(theta)*cos(phi+qX)+(RZIXY*cos(qZ)-RZIYY*sin(qZ))*(  ...
sin(qZ)*cos(theta)+sin(theta)*cos(phi)*cos(qZ))-RXIXZ*sin(theta)*sin(phi+qX)-(CIXX+RXIXX+mR*RCMZ^2+2*mR*(RCMY^2+1.5*RCMX^2))*cos(  ...
theta)-(RYIXZ*cos(qY)+RYIZZ*sin(qY))*(sin(qY)*cos(theta)+sin(phi)*sin(theta)*cos(qY))-(RYIXX*cos(qY)+RYIXZ*sin(qY))*(cos(qY)*cos(  ...
theta)-sin(phi)*sin(qY)*sin(theta))-(RZIXX*cos(qZ)-RZIXY*sin(qZ))*(cos(qZ)*cos(theta)-sin(qZ)*sin(theta)*cos(phi))-sin(phi)*sin(  ...
theta)*(CIXZ+mR*RCMX*RCMY+mR*RCMX^2+mR*RCMY*RCMZ+RZIXZ*cos(qZ)-RZIYZ*sin(qZ))-sin(theta)*cos(phi)*(mR*RCMX*RCMY+mR*RCMX*RCMZ+mR*RCMY*  ...
RCMZ-CIXY-RYIXY*cos(qY)-RYIYZ*sin(qY)))+(RXIXY*sin(phi+qX)+RXIXZ*cos(phi+qX)+cos(phi)*cos(qY)*(RYIXZ*cos(qY)+RYIZZ*sin(qY))+sin(phi)*  ...
sin(qZ)*(RZIXX*cos(qZ)-RZIXY*sin(qZ))+sin(phi)*cos(qZ)*(RZIXY*cos(qZ)-RZIYY*sin(qZ))+cos(phi)*(CIXZ+mR*RCMX*RCMY+mR*RCMX^2+mR*RCMY*  ...
RCMZ+RZIXZ*cos(qZ)-RZIYZ*sin(qZ))-sin(qY)*cos(phi)*(RYIXX*cos(qY)+RYIXZ*sin(qY))-sin(phi)*(mR*RCMX*RCMY+mR*RCMX*RCMZ+mR*RCMY*RCMZ-  ...
CIXY-RYIXY*cos(qY)-RYIYZ*sin(qY)))*(sin(theta)*sin(phi+qX)*(RXIYZ*sin(phi+qX)+RXIZZ*cos(phi+qX))+(cos(qZ)*cos(theta)-sin(qZ)*sin(  ...
theta)*cos(phi))*(RZIXZ*cos(phi)+RZIXX*sin(phi)*sin(qZ)+RZIXY*sin(phi)*cos(qZ))+sin(theta)*cos(phi)*(RYIXY*sin(qY)*cos(phi)-CIYY*  ...
sin(phi)-CIYZ*cos(phi)-RYIYY*sin(phi)-2*mR*RCMX*RCMY*cos(phi)-mR*RCMX*RCMZ*cos(phi)-RYIYZ*cos(phi)*cos(qY))+cos(theta)*(CIXY*sin(  ...
phi)+CIXZ*cos(phi)+RXIXY*sin(phi+qX)+RXIXZ*cos(phi+qX)+mR*RCMX*(RCMX*cos(phi)-RCMY*sin(phi))+mR*RCMY*(RCMX*cos(phi)-RCMZ*sin(phi))-  ...
mR*RCMZ*(RCMX*sin(phi)-RCMY*cos(phi)))-sin(theta)*cos(phi+qX)*(RXIYY*sin(phi+qX)+RXIYZ*cos(phi+qX))-(sin(qZ)*cos(theta)+sin(  ...
theta)*cos(phi)*cos(qZ))*(RZIYZ*cos(phi)+RZIXY*sin(phi)*sin(qZ)+RZIYY*sin(phi)*cos(qZ))-(sin(qY)*cos(theta)+sin(phi)*sin(theta)*cos(  ...
qY))*(RYIXZ*sin(qY)*cos(phi)-RYIYZ*sin(phi)-RYIZZ*cos(phi)*cos(qY))-(cos(qY)*cos(theta)-sin(phi)*sin(qY)*sin(theta))*(RYIXX*sin(qY)*  ...
cos(phi)-RYIXY*sin(phi)-RYIXZ*cos(phi)*cos(qY))-sin(phi)*sin(theta)*(mR*RCMX^2*cos(phi)-CIYZ*sin(phi)-CIZZ*cos(phi)-RZIZZ*cos(phi)-  ...
2*mR*RCMX*RCMY*sin(phi)-RZIXZ*sin(phi)*sin(qZ)-RZIYZ*sin(phi)*cos(qZ)-mR*RCMZ*(RCMX*sin(phi)+RCMZ*cos(phi)))));

end
